simulink model "travelling_wind_rectangle"  (R2019b)
settings: Solver=VariableStepAuto  StartTime=0.0  StopTime=10.0  RelTol=1e-3
values from neighbouring files (symbols this model uses):
  wind_amplitude = 1    [create_travelling_wind_rectangle.m]    (also in create_travelling_wind_sine.m; run_wheat_line_sway_experiment.m)
  wind_frequency = 2    [create_travelling_wind_rectangle.m]    (also in create_travelling_wind_sine.m = 5; run_wheat_line_sway_experiment.m = 50)
  wind_phase_cycle = 5    [create_travelling_wind_rectangle.m]    (also in create_travelling_wind_sine.m = 10; run_wheat_line_sway_experiment.m = 250)
settings Model: Creator=yz655  LastModifiedBy=yz655

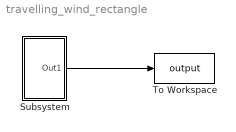
== system travelling_wind_rectangle ==
  Subsystem : Subsystem
  To Workspace : ToWorkspace  VariableName=output  SaveFormat=Timeseries  SampleTime=-1
  wires:
  Subsystem/1(Out1) -> To Workspace/1

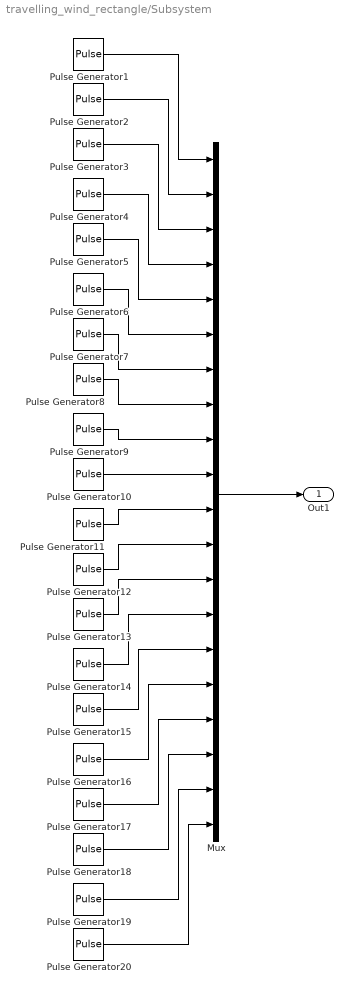
== system travelling_wind_rectangle/Subsystem ==
  Mux : Mux  Inputs=20
  Pulse Generator1 : DiscretePulseGenerator  PulseType=Time based  Amplitude=wind_amplitude  Period=1/wind_frequency  PulseWidth=50  PhaseDelay=1/wind_phase_cycle*1
  Pulse Generator10 : DiscretePulseGenerator  PulseType=Time based  Amplitude=wind_amplitude  Period=1/wind_frequency  PulseWidth=50  PhaseDelay=1/wind_phase_cycle*10
  Pulse Generator11 : DiscretePulseGenerator  PulseType=Time based  Amplitude=wind_amplitude  Period=1/wind_frequency  PulseWidth=50  PhaseDelay=1/wind_phase_cycle*11
  Pulse Generator12 : DiscretePulseGenerator  PulseType=Time based  Amplitude=wind_amplitude  Period=1/wind_frequency  PulseWidth=50  PhaseDelay=1/wind_phase_cycle*12
  Pulse Generator13 : DiscretePulseGenerator  PulseType=Time based  Amplitude=wind_amplitude  Period=1/wind_frequency  PulseWidth=50  PhaseDelay=1/wind_phase_cycle*13
  Pulse Generator14 : DiscretePulseGenerator  PulseType=Time based  Amplitude=wind_amplitude  Period=1/wind_frequency  PulseWidth=50  PhaseDelay=1/wind_phase_cycle*14
  Pulse Generator15 : DiscretePulseGenerator  PulseType=Time based  Amplitude=wind_amplitude  Period=1/wind_frequency  PulseWidth=50  PhaseDelay=1/wind_phase_cycle*15
  Pulse Generator16 : DiscretePulseGenerator  PulseType=Time based  Amplitude=wind_amplitude  Period=1/wind_frequency  PulseWidth=50  PhaseDelay=1/wind_phase_cycle*16
  Pulse Generator17 : DiscretePulseGenerator  PulseType=Time based  Amplitude=wind_amplitude  Period=1/wind_frequency  PulseWidth=50  PhaseDelay=1/wind_phase_cycle*17
  Pulse Generator18 : DiscretePulseGenerator  PulseType=Time based  Amplitude=wind_amplitude  Period=1/wind_frequency  PulseWidth=50  PhaseDelay=1/wind_phase_cycle*18
  Pulse Generator19 : DiscretePulseGenerator  PulseType=Time based  Amplitude=wind_amplitude  Period=1/wind_frequency  PulseWidth=50  PhaseDelay=1/wind_phase_cycle*19
  Pulse Generator2 : DiscretePulseGenerator  PulseType=Time based  Amplitude=wind_amplitude  Period=1/wind_frequency  PulseWidth=50  PhaseDelay=1/wind_phase_cycle*2
  Pulse Generator20 : DiscretePulseGenerator  PulseType=Time based  Amplitude=wind_amplitude  Period=1/wind_frequency  PulseWidth=50  PhaseDelay=1/wind_phase_cycle*20
  Pulse Generator3 : DiscretePulseGenerator  PulseType=Time based  Amplitude=wind_amplitude  Period=1/wind_frequency  PulseWidth=50  PhaseDelay=1/wind_phase_cycle*3
  Pulse Generator4 : DiscretePulseGenerator  PulseType=Time based  Amplitude=wind_amplitude  Period=1/wind_frequency  PulseWidth=50  PhaseDelay=1/wind_phase_cycle*4
  Pulse Generator5 : DiscretePulseGenerator  PulseType=Time based  Amplitude=wind_amplitude  Period=1/wind_frequency  PulseWidth=50  PhaseDelay=1/wind_phase_cycle*5
  Pulse Generator6 : DiscretePulseGenerator  PulseType=Time based  Amplitude=wind_amplitude  Period=1/wind_frequency  PulseWidth=50  PhaseDelay=1/wind_phase_cycle*6
  Pulse Generator7 : DiscretePulseGenerator  PulseType=Time based  Amplitude=wind_amplitude  Period=1/wind_frequency  PulseWidth=50  PhaseDelay=1/wind_phase_cycle*7
  Pulse Generator8 : DiscretePulseGenerator  PulseType=Time based  Amplitude=wind_amplitude  Period=1/wind_frequency  PulseWidth=50  PhaseDelay=1/wind_phase_cycle*8
  Pulse Generator9 : DiscretePulseGenerator  PulseType=Time based  Amplitude=wind_amplitude  Period=1/wind_frequency  PulseWidth=50  PhaseDelay=1/wind_phase_cycle*9
  Out1 : Outport
  wires:
  Pulse Generator17/1 -> Mux/17
  Pulse Generator18/1 -> Mux/18
  Pulse Generator6/1 -> Mux/6
  Pulse Generator19/1 -> Mux/19
  Pulse Generator16/1 -> Mux/16
  Pulse Generator13/1 -> Mux/13
  Pulse Generator20/1 -> Mux/20
  Pulse Generator14/1 -> Mux/14
  Pulse Generator12/1 -> Mux/12
  Pulse Generator15/1 -> Mux/15
  Pulse Generator11/1 -> Mux/11
  Pulse Generator10/1 -> Mux/10
  Pulse Generator9/1 -> Mux/9
  Pulse Generator8/1 -> Mux/8
  Pulse Generator7/1 -> Mux/7
  Pulse Generator5/1 -> Mux/5
  Pulse Generator4/1 -> Mux/4
  Pulse Generator3/1 -> Mux/3
  Pulse Generator2/1 -> Mux/2
  Pulse Generator1/1 -> Mux/1
  Mux/1 -> Out1/1
